simulink model "final_quadruped_060622_old"  (R2021a)
settings: Solver=ode15s  StartTime=0.0  StopTime=40  RelTol=1e-3  EnableMultiTasking=on
values from neighbouring files (symbols this model uses):
  foot_x = 8    [bipedparameters.m]    (also in fcn.m; finalrobotParameters.m; finalrobotParameters_110522.m; finalrobotParameters_140522.m)
  foot_y = 6    [bipedparameters.m]    (also in fcn.m; finalrobotParameters.m; finalrobotParameters_110522.m; finalrobotParameters_140522.m)
  foot_z = 1    [bipedparameters.m]    (also in fcn.m; finalrobotParameters.m; finalrobotParameters_110522.m; finalrobotParameters_140522.m)
  height_plane = 0.025    [bipedparameters.m]    (also in finalrobotParameters.m; finalrobotParameters_110522.m; finalrobotParameters_140522.m; finalrobotParameters_240522.m)
  kd = 1000    [bipedparameters.m]    (also in finalrobotParameters_140522.m = 5; finalrobotParameters_240522.m)
  ki = 1000    [bipedparameters.m]    (also in finalrobotParameters_140522.m = 5; finalrobotParameters_240522.m)
  kp = 1000    [bipedparameters.m]    (also in finalrobotParameters_140522.m = 5; finalrobotParameters_240522.m)
  lower_leg_length = 10    [bipedparameters.m]    (also in fcn.m; finalrobotParameters.m; finalrobotParameters_110522.m; finalrobotParameters_140522.m)
  m_ll = density*leg_radius*leg_radius*lower_leg_length*3.141592653589*0.01*0.01*0.01    (= 0.0176714586764)    [bipedparameters.m]    (also in fcn.m; finalrobotParameters_140522.m; finalrobotParameters_240522.m; hdotlb.m)
  m_ul = density*leg_radius*leg_radius*upper_leg_length*3.141592653589*0.01*0.01*0.01    (= 0.0176714586764)    [bipedparameters.m]    (also in fcn.m; finalrobotParameters_140522.m; finalrobotParameters_240522.m; hdotlb.m)
  plane_x = 25    [bipedparameters.m]    (also in finalrobotParameters.m; finalrobotParameters_110522.m; finalrobotParameters_140522.m; finalrobotParameters_240522.m)
  plane_y = 3    [bipedparameters.m]    (also in finalrobotParameters.m; finalrobotParameters_110522.m; finalrobotParameters_140522.m; finalrobotParameters_240522.m)
  torso_offset_x = -0.5    [bipedparameters.m]    (also in finalrobotParameters.m = 10; finalrobotParameters_110522.m = 10; finalrobotParameters_140522.m = 10; finalrobotParameters_240522.m = 10)
  torso_offset_z = -2    [bipedparameters.m]    (also in finalrobotParameters.m; finalrobotParameters_110522.m; finalrobotParameters_140522.m; finalrobotParameters_240522.m)
  torso_x = 5    [bipedparameters.m]    (also in fcn.m = 25; finalrobotParameters.m = 25; finalrobotParameters_110522.m = 25; finalrobotParameters_140522.m = 25)
  torso_y = 10    [bipedparameters.m]    (also in fcn.m = 16; finalrobotParameters.m = 16; finalrobotParameters_110522.m = 16; finalrobotParameters_140522.m = 16)
  torso_z = 8    [bipedparameters.m]    (also in fcn.m = 10; finalrobotParameters.m = 10; finalrobotParameters_110522.m = 10; finalrobotParameters_140522.m = 10)
  upper_leg_length = 10    [bipedparameters.m]    (also in fcn.m; finalrobotParameters.m; finalrobotParameters_110522.m; finalrobotParameters_140522.m)
undefined symbols (not defined in the file or in its folder): angleLFknee, speedLFknee, torqueLFknee, X, Y, Z
libraries: nesl_utility x93, sm_lib x71, Contact_Forces_Lib x16, pid_lib x12, fl_lib x3
(part 6 of 6)

== matlab function final_quadruped_060622_old/Model/Right Leg Back/MATLAB Function2 ==
  data: tddRB input; tddRB_hip output; tddRB_knee output; tddRB_ankle output
function [tddRB_hip, tddRB_knee, tddRB_ankle] = fcn(tddRB)
tddRB_hip=tddRB(1);
tddRB_knee=tddRB(2);
tddRB_ankle=tddRB(3);
end

== matlab function final_quadruped_060622_old/Model/Left LegBack/MATLAB Function2 ==
  data: tddLB input; tddLB_hip output; tddLB_knee output; tddLB_ankle output
function [tddLB_hip, tddLB_knee, tddLB_ankle] = fcn(tddLB)
tddLB_hip=tddLB(1);
tddLB_knee=tddLB(2);
tddLB_ankle=tddLB(3);
end

== matlab function final_quadruped_060622_old/Subsystem/MATLAB Function4 ==
  data: vx input; vy input; v output; vz input
function v = fcn(vx,vy,vz)
v=[vx;vy;vz];
end

== matlab function final_quadruped_060622_old/Subsystem/MATLAB Function5 ==
  data: vx input; vy input; v output; vz input
function v = fcn(vx,vy,vz)
v=[vx;vy;vz];
end

== matlab function final_quadruped_060622_old/Subsystem/MATLAB Function6 ==
  data: vx input; vy input; v output; vz input
function v = fcn(vx,vy,vz)
v=[vx;vy;vz];
end

== matlab function final_quadruped_060622_old/Subsystem/MATLAB Function7 ==
  data: vx input; vy input; v output; vz input
function v = fcn(vx,vy,vz)
v=[vx;vy;vz];
end

== matlab function final_quadruped_060622_old/Subsystem/MATLAB Function13 ==
  data: vulRF input; vllRF input; Mvcm output; vfRF input; vulLF input; vllLF input; vfLF input; vulRB input; vllRB input; vfRB input; vulLB input; vllLB input; vfLB input; v_torso input
function Mvcm = fcn(vulRF,vllRF,vfRF,vulLF,vllLF,vfLF,vulRB,vllRB,vfRB,vulLB,vllLB,vfLB,v_torso)
%%
lower_leg_length = 10;
upper_leg_length = 10;
density = 1000;
foot_density=2000;
leg_radius = 0.75;
foot_x = 8;
foot_y = 6;
foot_z = 1;
torso_y = 16;
torso_x = 25;
torso_z = 10;
m_ul=density*leg_radius*leg_radius*upper_leg_length*3.141592653589*0.01*0.01*0.01;
m_ll=density*leg_radius*leg_radius*lower_leg_length*3.141592653589*0.01*0.01*0.01;
m_foot=foot_density*foot_x*foot_y*foot_z*0.000001;
m_torso=density*torso_x*torso_y*torso_z*0.000001;
%%
Mvcm=m_torso*v_torso+(m_ul*vulRF+m_ll*vllRF+m_foot*vfRF)+(m_ul*vulLF+m_ll*vllLF+m_foot*vfLF)+(m_ul*vulRB+m_ll*vllRB+m_foot*vfRB)+(m_ul*vulLB+m_ll*vllLB+m_foot*vfLB);
end

== matlab function final_quadruped_060622_old/Subsystem/MATLAB Function8 ==
  data: vx input; vy input; v output; vz input
function v = fcn(vx,vy,vz)
v=[vx;vy;vz];
end

== matlab function final_quadruped_060622_old/Subsystem/MATLAB Function9 ==
  data: vx input; vy input; v output; vz input
function v = fcn(vx,vy,vz)
v=[vx;vy;vz];
end

== matlab function final_quadruped_060622_old/Subsystem/MATLAB Function10 ==
  data: vx input; vy input; v output; vz input
function v = fcn(vx,vy,vz)
v=[vx;vy;vz];
end

== matlab function final_quadruped_060622_old/Subsystem/MATLAB Function11 ==
  data: vx input; vy input; v output; vz input
function v = fcn(vx,vy,vz)
v=[vx;vy;vz];
end

== matlab function final_quadruped_060622_old/Subsystem/MATLAB Function12 ==
  data: vx input; vy input; v output; vz input
function v = fcn(vx,vy,vz)
v=[vx;vy;vz];
end

== matlab function final_quadruped_060622_old/Subsystem/MATLAB Function14 ==
  data: vx input; vy input; v output; vz input
function v = fcn(vx,vy,vz)
v=[vx;vy;vz];
end

== matlab function final_quadruped_060622_old/Model/Right Leg Front /MATLAB Function ==
  data: ankle input; knee input; tdRF output; hip input
function tdRF= fcn(ankle, knee, hip)
tdRF=[hip;knee;ankle];
end

== matlab function final_quadruped_060622_old/Model/Left Leg Front/MATLAB Function ==
  data: ankle input; knee input; tdRF output; hip input
function tdRF= fcn(ankle, knee, hip)
tdRF=[hip;knee;ankle];
end

== matlab function final_quadruped_060622_old/Model/Right Leg Back/MATLAB Function ==
  data: ankle input; knee input; tdRF output; hip input
function tdRF= fcn(ankle, knee, hip)
tdRF=[hip;knee;ankle];
end

== matlab function final_quadruped_060622_old/Model/Left LegBack/MATLAB Function ==
  data: ankle input; knee input; tdRF output; hip input
function tdRF= fcn(ankle, knee, hip)
tdRF=[hip;knee;ankle];
end

== matlab function final_quadruped_060622_old/Model/MATLAB Function ==
  data: tdRF input; td output; tdLF input; tdRB input; tdLB input
function td = fcn(tdRF,tdLF,tdRB,tdLB)
td=[tdRF;tdLF;tdRB;tdLB];
end

== matlab function final_quadruped_060622_old/Model/MATLAB Function1 ==
  data: h input; htd output; td input
function htd = fcn(h, td)
htd=h*td;
end

== matlab function final_quadruped_060622_old/MATLAB Function1 ==
  data: Mvcm input; error output; htd input; v_torso input
function error = fcn(Mvcm,htd, v_torso)
%%
lower_leg_length = 10;
upper_leg_length = 10;
density = 1000;
foot_density=2000;
leg_radius = 0.75;
foot_x = 8;
foot_y = 6;
foot_z = 1;
torso_y = 16;
torso_x = 25;
torso_z = 10;
m_ul=density*leg_radius*leg_radius*upper_leg_length*3.141592653589*0.01*0.01*0.01;
m_ll=density*leg_radius*leg_radius*lower_leg_length*3.141592653589*0.01*0.01*0.01;
m_foot=foot_density*foot_x*foot_y*foot_z*0.000001;
m_torso=density*torso_x*torso_y*torso_z*0.000001;
M=m_torso+(4*(m_ul+m_ll+m_foot));
%%
error=htd+M*v_torso-Mvcm;
end

== matlab function final_quadruped_060622_old/Subsystem/MATLAB Function2 ==
  data: vx input; vy input; v output; vz input
function v = fcn(vx,vy,vz)
v=[vx;vy;vz];
end

== matlab function final_quadruped_060622_old/Subsystem/MATLAB Function3 ==
  data: vx input; vy input; v output; vz input
function v = fcn(vx,vy,vz)
v=[vx;vy;vz];
end

== matlab function final_quadruped_060622_old/Model/Right Leg Front /Subsystem/MATLAB Function ==
  data: ea1g output; ea2g output; ea3g output; qha input; qaa input; Qquat input; qka input; aa1g output; aa2g output; cma1g output; cma2g output; cma3g output
function [ea1g,ea2g,ea3g,aa1g,aa2g,cma1g,cma2g,cma3g] = fcn(qha,qaa,Qquat,qka)
%%
lower_leg_length = 10;
upper_leg_length = 10;
foot_offset=[-1; 0; 0];

%%
disp(Qquat);
Qquat
Qd0g=quat2rotm([Qquat(1) Qquat(2) Qquat(3) Qquat(4)]);
Qd10=[cos(qha) 0 sin(qha);
      0 1 0 ;
      -sin(qha) 0 cos(qha)];
Qd1g=Qd10*Qd0g;
  
Qd21=[cos(qka) 0 sin(qka);
      0 1 0 ;
      -sin(qka) 0 cos(qka)];
  
Qd32=[1 0 0;
      0 cos(qaa) -sin(qaa);
      0 sin(qaa) cos(qaa)];
  
Qd20 = Qd21* Qd10;
Qd30=Qd32*Qd20;
Qd2g=Qd20*Qd0g;
Qd3g=Qd30*Qd0g;

%axis in local frames
ed1l=[0;
      1;
      0];
ed2l=[0;
      1;
      0];
ed3l=[0;
     0;
     1];
  
%link vector in local frame
ad1l=[0;
      0;
      -upper_leg_length];
   
ad2l=[0;
      0;
      -lower_leg_length];
         
%axis in global frames
ea1g = Qd1g*ed1l;
ea2g = Qd2g*ed2l;
ea3g = Qd3g*ed3l;

%link vector in global frame
aa1g = Qd1g*ad1l;
aa2g = Qd2g*ad2l;

%COM distances in base frame
cma1g=aa1g/2;
cma2g=aa2g/2;
cma3g=Qd3g*foot_offset;


end

== matlab function final_quadruped_060622_old/Model/Left Leg Front/Subsystem/MATLAB Function ==
  data: eb1g output; eb2g output; eb3g output; qhb input; qab input; Qquat input; qkb input; ab1g output; ab2g output; cmb1g output; cmb2g output; cmb3g output
function [eb1g,eb2g,eb3g,ab1g,ab2g,cmb1g,cmb2g,cmb3g] = fcn(qhb,qab,Qquat,qkb)
%%
lower_leg_length = 10;
upper_leg_length = 10;
foot_offset=[-1; 0; 0];

%%
Qd10=zeros(3,3);
% disp(Qquat);
% Qquat=reshape(Qquat,4,1);
Qquat;
Qd0g=quat2rotm([Qquat(1) Qquat(2) Qquat(3) Qquat(4)]);
% Qd0geul=quat2eul(Qquat);
% Qd0g=eul2rotm(Qd0geul);
Qd10=[cos(qhb) 0 sin(qhb);
      0 1 0 ;
      -sin(qhb) 0 cos(qhb)];
Qd1g=Qd10*Qd0g;
  
Qd21=[cos(qkb) 0 sin(qkb);
      0 1 0 ;
      -sin(qkb) 0 cos(qkb)];
  
Qd32=[1 0 0;
      0 cos(qab) -sin(qab);
      0 sin(qab) cos(qab)];
  
Qd20 = Qd21* Qd10;
Qd30=Qd32*Qd20;
Qd2g=Qd20*Qd0g;
Qd3g=Qd30*Qd0g;

%axis in local frames
ed1l=[0;
      1;
      0];
ed2l=[0;
      1;
      0];
ed3l=[0;
     0;
     1];
  
%link vector in local frame
ad1l=[0;
      0;
      -upper_leg_length];
   
ad2l=[0;
      0;
      -lower_leg_length];
         
%axis in global frames
eb1g = Qd1g*ed1l;
eb2g = Qd2g*ed2l;
eb3g = Qd3g*ed3l;

%link vector in global frame
ab1g = Qd1g*ad1l;
ab2g = Qd2g*ad2l;

%COM distances in base frame
cmb1g=ab1g/2;
cmb2g=ab2g/2;
cmb3g=Qd3g*foot_offset;


end

== matlab function final_quadruped_060622_old/Model/Right Leg Back/Subsystem/MATLAB Function ==
  data: ec1g output; ec2g output; ec3g output; qhc input; qac input; Qquat input; qkc input; ac1g output; ac2g output; cmc1g output; cmc2g output; cmc3g output
function [ec1g,ec2g,ec3g,ac1g,ac2g,cmc1g,cmc2g,cmc3g] = fcn(qhc,qac,Qquat,qkc)
%%
lower_leg_length = 10;
upper_leg_length = 10;
foot_offset=[-1; 0; 0];

%%
Qd0g=quat2rotm([Qquat(1) Qquat(2) Qquat(3) Qquat(4)]);
Qd10=[cos(qhc) 0 sin(qhc);
      0 1 0 ;
      -sin(qhc) 0 cos(qhc)];
Qd1g=Qd10*Qd0g;
  
Qd21=[cos(qkc) 0 sin(qkc);
      0 1 0 ;
      -sin(qkc) 0 cos(qkc)];
  
Qd32=[1 0 0;
      0 cos(qac) -sin(qac);
      0 sin(qac) cos(qac)];
  
Qd20 = Qd21* Qd10;
Qd30=Qd32*Qd20;
Qd2g=Qd20*Qd0g;
Qd3g=Qd30*Qd0g;

%axis in local frames
ed1l=[0;
      1;
      0];
ed2l=[0;
      1;
      0];
ed3l=[0;
     0;
     1];
  
%link vector in local frame
ad1l=[0;
      0;
      -upper_leg_length];
   
ad2l=[0;
      0;
      -lower_leg_length];
         
%axis in global frames
ec1g = Qd1g*ed1l;
ec2g = Qd2g*ed2l;
ec3g = Qd3g*ed3l;

%link vector in global frame
ac1g = Qd1g*ad1l;
ac2g = Qd2g*ad2l;

%COM distances in base frame
cmc1g=ac1g/2;
cmc2g=ac2g/2;
cmc3g=Qd3g*foot_offset;


end
